simulink library "lib_Convection_NonDimParms"  (R2015a)
settings: Solver=ode45  StartTime=0.0  StopTime=10.0  RelTol=1e-3
settings Model: Creator=jlkratz  LastModifiedBy=jlkratz

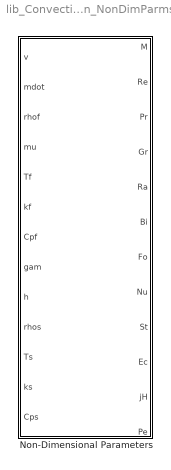
== system lib_Convection_NonDimParms ==
  Non-Dimensional Parameters : Subsystem  mask(TSAT: Non-Dimensional Parameters Block){M_M=on, Re_M=on, Pr_M=on, Gr_M=on, Ra_M=on, Bi_M=on, Fo_M=on, Nu_M=on, St_M=on, Ec_M=on, jH_M=on, Pe_M=on, perfGas_M=on, R_M=1716, mdot_A_or_rhov_M=on, A_M=1, L_M=1, g_M=32.174, t_M=1, BN_M=double(gcb)}
      mask prompts: M_M "M_M - Mach Number"; Re_M "Re_M - Reynolds Number"; Pr_M "Pr_M - Prandtl Number"; Gr_M "Gr_M - Grashof Number"; Ra_M "Ra_M - Rayliegh Number"; Bi_M "Bi_M - Biot Number"; Fo_M "Fo_M - Fourier Number"; Nu_M "Nu_M - Nusselt Number"; St_M "St_M - Stanton Number"; Ec_M "Ec_M - Eckert Number"; jH_M "jH_M - Colburn j facotr"; Pe_M "Pe_M - Peclet Number"; perfGas_M "perfGas_M - Perfect gas?"; R_M "R_M - Real gas constant"; mdot_A_or_rhov_M "mdot_A_or_rhov_M - Compute Re using mass flow rate or velocity (checked mdot, unchecked v)?"; A_M "A_M - Flow area"; L_M "L_M - Characteristic length"; g_M "g_M - Acceleration due to gravity"; t_M "t_M - Charateristic time-scale"; BN_M "BN_M - Block Name"
      mask help:
      | This block computes various non-dimensional quanties that are related to heat transfer. See the block help menu for a full description of the non-dimensional parameters addressed in this block and definitions of all of the inputs and parameters.
      |
      | This block can accept inputs of any dimensions as long as they are all consistent. Any units can be used in the inputs and parameters as long as they are consistent and on a total scale (no relative values and no units of a non-total scale. Ex. no degrees Celsius and Farhenhiet).
      mask init:
      | % Setup inports ----------------------------------------------------------%
      | 
      | % Inport Numbers
      | n = 1; %first inport
      | 
      | % Velocity
      | if M_M == 1 || (Re_M == 1 && mdot_A_or_rhov_M == 0) || Pe_M == 1 || Ec_M == 1 || St_M == 1
      |     if strcmp(get_param([BN_M '/v'],'BlockType'),'Constant')
      |         MSK_ReplaceBlock_TSAT([BN_M '/v'],'built-in/Inport');
      |     end
      |     set_param([BN_M '/v'],'Port',num2str(n));
      |     n = n + 1;
      | else
      |     if strcmp(get_param([BN_M '/v'],'BlockType'),'Inport')
      |         MSK_ReplaceBlock_TSAT([BN_M '/v'],'built-in/Constant');
      |         set_param([BN_M '/v'],'Value','10');
      |     end
      | end
      | 
      | % Mass Flow Rate
      | if (Re_M == 1 && mdot_A_or_rhov_M == 1)
      |     if strcmp(get_param([BN_M '/mdot'],'BlockType'),'Constant')
      |         MSK_ReplaceBlock_TSAT([BN_M '/mdot'],'built-in/Inport');
      |     end
      |     set_param([BN_M '/mdot'],'Port',num2str(n));
      |     n = n + 1;
      | else
      |     if strcmp(get_param([BN_M '/mdot'],'BlockType'),'Inport')
      |         MSK_ReplaceBlock_TSAT([BN_M '/mdot'],'built-in/Constant');
      |         set_param([BN_M '/mdot'],'Value','1');
      |     end
      | end
      | 
      | % Density of fluid
      | if (Re_M == 1 && mdot_A_or_rhov_M == 0) || Pe_M == 1 || St_M == 1 || Gr_M == 1 || Ra_M == 1
      |     if strcmp(get_param([BN_M '/rhof'],'BlockType'),'Constant')
      |         MSK_ReplaceBlock_TSAT([BN_M '/rhof'],'built-in/Inport');
      |     end
      |     set_param([BN_M '/rhof'],'Port',num2str(n));
      |     n = n + 1;
      | else
      |     if strcmp(get_param([BN_M '/rhof'],'BlockType'),'Inport')
      |         MSK_ReplaceBlock_TSAT([BN_M '/rhof'],'built-in/Constant');
      |         set_param([BN_M '/rhof'],'Value','0.00237');
      |     end
      | end
      | 
      | % Viscosity
      | if Re_M == 1 || Pr_M == 1 || Gr_M == 1 || Ra_M == 1 || jH_M == 1
      |     if strcmp(get_param([BN_M '/mu'],'BlockType'),'Constant')
      |         MSK_ReplaceBlock_TSAT([BN_M '/mu'],'built-in/Inport');
      |     end
      |     set_param([BN_M '/mu'],'Port',num2str(n));
      |     n = n + 1;
      | else
      |     if strcmp(get_param([BN_M '/mu'],'BlockType'),'Inport')
      |         MSK_ReplaceBlock_TSAT([BN_M '/mu'],'built-in/Constant');
      |         set_param([BN_M '/mu'],'Value','0.0000005');
      |     end
      | end
      | 
      | % Temperature of fluid
      | if Gr_M == 1 || Ra_M == 1 || Ec_M == 1 || (M_M == 1 && perfGas_M == 1)
      |     if strcmp(get_param([BN_M '/Tf'],'BlockType'),'Constant')
      |         MSK_ReplaceBlock_TSAT([BN_M '/Tf'],'built-in/Inport');
      |     end
      |     set_param([BN_M '/Tf'],'Port',num2str(n));
      |     n = n + 1;
      | else
      |     if strcmp(get_param([BN_M '/Tf'],'BlockType'),'Inport')
      |         MSK_ReplaceBlock_TSAT([BN_M '/Tf'],'built-in/Constant');
      |         set_param([BN_M '/Tf'],'Value','0.0000005');
      |     end
      | end
      | 
      | % Thermal conductivity of fluid
      | if Pr_M == 1 || Nu_M == 1 || Pe_M == 1
      |     if strcmp(get_param([BN_M '/kf'],'BlockType'),'Constant')
      |         MSK_ReplaceBlock_TSAT([BN_M '/kf'],'built-in/Inport');
      |     end
      |     set_param([BN_M '/kf'],'Port',num2str(n));
      |     n = n + 1;
      | else
      |     if strcmp(get_param([BN_M '/kf'],'BlockType'),'Inport')
      |         MSK_ReplaceBlock_TSAT([BN_M '/kf'],'built-in/Constant');
      |         set_param([BN_M '/kf'],'Value','0.00000413');
      |     end
      | end
      | 
      | % Heat Capacity of fluid
      | if Pr_M == 1 || Ec_M == 1 || Pe_M == 1 || St_M == 1
      |     if strcmp(get_param([BN_M '/Cpf'],'BlockType'),'Constant')
      |         MSK_ReplaceBlock_TSAT([BN_M '/Cpf'],'built-in/Inport');
      |     end
      |     set_param([BN_M '/Cpf'],'Port',num2str(n));
      |     n = n + 1;
      | else
      |     if strcmp(get_param([BN_M '/Cpf'],'BlockType'),'Inport')
      |         MSK_ReplaceBlock_TSAT([BN_M '/Cpf'],'built-in/Constant');
      |         set_param([BN_M '/Cpf'],'Value','7.72');
      |     end
      | end
      | 
      | % Specific heat ratio
      | if (M_M == 1 && perfGas_M == 1)
      |     if strcmp(get_param([BN_M '/gam'],'BlockType'),'Constant')
      |         MSK_ReplaceBlock_TSAT([BN_M '/gam'],'built-in/Inport');
      |     end
      |     set_param([BN_M '/gam'],'Port',num2str(n));
      |     n = n + 1;
      | else
      |     if strcmp(get_param([BN_M '/gam'],'BlockType'),'Inport')
      |         MSK_ReplaceBlock_TSAT([BN_M '/gam'],'built-in/Constant');
      |         set_param([BN_M '/gam'],'Value','1.4');
      |     end
      | end
      | 
      | % Convective heat transfer coefficient
      | if Bi_M == 1 || Nu_M == 1 || St_M == 1
      |     if strcmp(get_param([BN_M '/h'],'BlockType'),'Constant')
      |         MSK_ReplaceBlock_TSAT([BN_M '/h'],'built-in/Inport');
      |     end
      |     set_param([BN_M '/h'],'Port',num2str(n));
      |     n = n + 1;
      | else
      |     if strcmp(get_param([BN_M '/h'],'BlockType'),'Inport')
      |         MSK_ReplaceBlock_TSAT([BN_M '/h'],'built-in/Constant');
      |         set_param([BN_M '/h'],'Value','0.003');
      |     end
      | end
      | 
      | % Speed of sound
      | if (M_M == 1 && perfGas_M == 0)
      |     if strcmp(get_param([BN_M '/a'],'BlockType'),'Constant')
      |         MSK_ReplaceBlock_TSAT([BN_M '/a'],'built-in/Inport');
      |     end
      |     set_param([BN_M '/a'],'Port',num2str(n));
      |     n = n + 1;
      | else
      |     if strcmp(get_param([BN_M '/a'],'BlockType'),'Inport')
      |         MSK_ReplaceBlock_TSAT([BN_M '/a'],'built-in/Constant');
      |         set_param([BN_M '/a'],'Value','1125.33');
      |     end
      | end
      | 
      | % Expansion coefficient
      | if (Gr_M == 1 && perfGas_M == 0) || (Ra_M == 1 && perfGas_M == 0)
      |     if strcmp(get_param([BN_M '/beta'],'BlockType'),'Constant')
      |         MSK_ReplaceBlock_TSAT([BN_M '/beta'],'built-in/Inport');
      |     end
      |     set_param([BN_M '/beta'],'Port',num2str(n));
      |     n = n + 1;
      | else
      |     if strcmp(get_param([BN_M '/beta'],'BlockType'),'Inport')
      |         MSK_ReplaceBlock_TSAT([BN_M '/beta'],'built-in/Constant');
      |         set_param([BN_M '/beta'],'Value','0.002');
      |     end
      | end
      | 
      | % Density of solid (body)
      | if Fo_M == 1
      |     if strcmp(get_param([BN_M '/rhos'],'BlockType'),'Constant')
      |         MSK_ReplaceBlock_TSAT([BN_M '/rhos'],'built-in/Inport');
      |     end
      |     set_param([BN_M '/rhos'],'Port',num2str(n));
      |     n = n + 1;
      | else
      |     if strcmp(get_param([BN_M '/rhos'],'BlockType'),'Inport')
      |         MSK_ReplaceBlock_TSAT([BN_M '/rhos'],'built-in/Constant');
      |         set_param([BN_M '/rhos'],'Value','2');
      |     end
      | end
      | 
      | % Temperature of solid (body)
      | if Gr_M == 1 || Ra_M == 1 || Ec_M == 1
      |     if strcmp(get_param([BN_M '/Ts'],'BlockType'),'Constant')
      |         MSK_ReplaceBlock_TSAT([BN_M '/Ts'],'built-in/Inport');
      |     end
      |     set_param([BN_M '/Ts'],'Port',num2str(n));
      |     n = n + 1;
      | else
      |     if strcmp(get_param([BN_M '/Ts'],'BlockType'),'Inport')
      |         MSK_ReplaceBlock_TSAT([BN_M '/Ts'],'built-in/Constant');
      |         set_param([BN_M '/Ts'],'Value','1000');
      |     end
      | end
      | 
      | % Thermal conductivity of solid (body)
      | if Fo_M == 1 || Bi_M == 1
      |     if strcmp(get_param([BN_M '/ks'],'BlockType'),'Constant')
      |         MSK_ReplaceBlock_TSAT([BN_M '/ks'],'built-in/Inport');
      |     end
      |     set_param([BN_M '/ks'],'Port',num2str(n));
      |     n = n + 1;
      | else
      |     if strcmp(get_param([BN_M '/ks'],'BlockType'),'Inport')
      |         MSK_ReplaceBlock_TSAT([BN_M '/ks'],'built-in/Constant');
      |         set_param([BN_M '/ks'],'Value','0.005');
      |     end
      | end
      | 
      | % Heat Capacity of solid (body)
      | if Fo_M == 1
      |     if strcmp(get_param([BN_M '/Cps'],'BlockType'),'Constant')
      |         MSK_ReplaceBlock_TSAT([BN_M '/Cps'],'built-in/Inport');
      |     end
      |     set_param([BN_M '/Cps'],'Port',num2str(n));
      |     n = n + 1;
      | else
      |     if strcmp(get_param([BN_M '/Cps'],'BlockType'),'Inport')
      |         MSK_ReplaceBlock_TSAT([BN_M '/Cps'],'built-in/Constant');
      |         set_param([BN_M '/Cps'],'Value','3.2');
      |     end
      | end
      | 
      | %Setup outports ----------------------------------------------------------%
      | 
      | % Outport Numbers
      | N = 1; %first outport
      | 
      | % Mach number
      | if M_M == 1
      |     if strcmp(get_param([BN_M '/M'],'BlockType'),'Terminator')
      |         MSK_ReplaceBlock_TSAT([BN_M '/M'],'built-in/Outport');
      |     end
      |     set_param([BN_M '/M'],'Port',num2str(N));
      |     N = N + 1;
      | elseif M_M == 0
      |     if strcmp(get_param([BN_M '/M'],'BlockType'),'Outport')
      |         MSK_ReplaceBlock_TSAT([BN_M '/M'],'built-in/Terminator');
      |     end
      | end
      | 
      | % Reynolds number
      | if Re_M == 1
      |     if strcmp(get_param([BN_M '/Re'],'BlockType'),'Terminator')
      |         MSK_ReplaceBlock_TSAT([BN_M '/Re'],'built-in/Outport');
      |     end
      |     set_param([BN_M '/Re'],'Port',num2str(N));
      |     N = N + 1;
      | elseif Re_M == 0
      |     if strcmp(get_param([BN_M '/Re'],'BlockType'),'Outport')
      |         MSK_ReplaceBlock_TSAT([BN_M '/Re'],'built-in/Terminator');
      |     end
      | end
      | 
      | % Prantdl number
      | if Pr_M == 1
      |     if strcmp(get_param([BN_M '/Pr'],'BlockType'),'Terminator')
      |         MSK_ReplaceBlock_TSAT([BN_M '/Pr'],'built-in/Outport');
      |     end
      |     set_param([BN_M '/Pr'],'Port',num2str(N));
      |     N = N + 1;
      | elseif Pr_M == 0
      |     if strcmp(get_param([BN_M '/Pr'],'BlockType'),'Outport')
      |         MSK_ReplaceBlock_TSAT([BN_M '/Pr'],'built-in/Terminator');
      |     end
      | end
      | 
      | % Grashof number
      | if Gr_M == 1
      |     if strcmp(get_param([BN_M '/Gr'],'BlockType'),'Terminator')
      |         MSK_ReplaceBlock_TSAT([BN_M '/Gr'],'built-in/Outport');
      |     end
      |     set_param([BN_M '/Gr'],'Port',num2str(N));
      |     N = N + 1;
      | elseif Gr_M == 0
      |     if strcmp(get_param([BN_M '/Gr'],'BlockType'),'Outport')
      |         MSK_ReplaceBlock_TSAT([BN_M '/Gr'],'built-in/Terminator');
      |     end
      | end
      | 
      | % Rayliegh number
      | if Ra_M == 1
      |     if strcmp(get_param([BN_M '/Ra'],'BlockType'),'Terminator')
      |         MSK_ReplaceBlock_TSAT([BN_M '/Ra'],'built-in/Outport');
      |     end
      |     set_param([BN_M '/Ra'],'Port',num2str(N));
      |     N = N + 1;
      | elseif Ra_M == 0
      |     if strcmp(get_param([BN_M '/Ra'],'BlockType'),'Outport')
      |         MSK_ReplaceBlock_TSAT([BN_M '/Ra'],'built-in/Terminator');
      |     end
      | end
      | 
      | % Biot number
      | if Bi_M == 1
      |     if strcmp(get_param([BN_M '/Bi'],'BlockType'),'Terminator')
      |         MSK_ReplaceBlock_TSAT([BN_M '/Bi'],'built-in/Outport');
      |     end
      |     set_param([BN_M '/Bi'],'Port',num2str(N));
      |     N = N + 1;
      | elseif Bi_M == 0
      |     if strcmp(get_param([BN_M '/Bi'],'BlockType'),'Outport')
      |         MSK_ReplaceBlock_TSAT([BN_M '/Bi'],'built-in/Terminator');
      |     end
      | end
      | 
      | % Fourier number
      | if Fo_M == 1
      |     if strcmp(get_param([BN_M '/Fo'],'BlockType'),'Terminator')
      |         MSK_ReplaceBlock_TSAT([BN_M '/Fo'],'built-in/Outport');
      |     end
      |     set_param([BN_M '/Fo'],'Port',num2str(N));
      |     N = N + 1;
      | elseif Fo_M == 0
      |     if strcmp(get_param([BN_M '/Fo'],'BlockType'),'Outport')
      |         MSK_ReplaceBlock_TSAT([BN_M '/Fo'],'built-in/Terminator');
      |     end
      | end
      | 
      | % Nusselt Number
      | if Nu_M == 1
      |     if strcmp(get_param([BN_M '/Nu'],'BlockType'),'Terminator')
      |         MSK_ReplaceBlock_TSAT([BN_M '/Nu'],'built-in/Outport');
      |     end
      |     set_param([BN_M '/Nu'],'Port',num2str(N));
      |     N = N + 1;
      | elseif Nu_M == 0
      |     if strcmp(get_param([BN_M '/Nu'],'BlockType'),'Outport')
      |         MSK_ReplaceBlock_TSAT([BN_M '/Nu'],'built-in/Terminator');
      |     end
      | end
      | 
      | % Stanton Number
      | if St_M == 1
      |     if strcmp(get_param([BN_M '/St'],'BlockType'),'Terminator')
      |         MSK_ReplaceBlock_TSAT([BN_M '/St'],'built-in/Outport');
      |     end
      |     set_param([BN_M '/St'],'Port',num2str(N));
      |     N = N + 1;
      | elseif St_M == 0
      |     if strcmp(get_param([BN_M '/St'],'BlockType'),'Outport')
      |         MSK_ReplaceBlock_TSAT([BN_M '/St'],'built-in/Terminator');
      |     end
      | end
      | 
      | % Eckert Number
      | if Ec_M == 1
      |     if strcmp(get_param([BN_M '/Ec'],'BlockType'),'Terminator')
      |         MSK_ReplaceBlock_TSAT([BN_M '/Ec'],'built-in/Outport');
      |     end
      |     set_param([BN_M '/Ec'],'Port',num2str(N));
      |     N = N + 1;
      | elseif Ec_M == 0
      |     if strcmp(get_param([BN_M '/Ec'],'BlockType'),'Outport')
      |         MSK_ReplaceBlock_TSAT([BN_M '/Ec'],'built-in/Terminator');
      |     end
      | end
      | 
      | % Colburn j factor
      | if jH_M == 1
      |     if strcmp(get_param([BN_M '/jH'],'BlockType'),'Terminator')
      |         MSK_ReplaceBlock_TSAT([BN_M '/jH'],'built-in/Outport');
      |     end
      |     set_param([BN_M '/jH'],'Port',num2str(N));
      |     N = N + 1;
      | elseif jH_M == 0
      |     if strcmp(get_param([BN_M '/jH'],'BlockType'),'Outport')
      |         MSK_ReplaceBlock_TSAT([BN_M '/jH'],'built-in/Terminator');
      |     end
      | end
      | 
      | % Peclet number
      | if Pe_M == 1
      |     if strcmp(get_param([BN_M '/Pe'],'BlockType'),'Terminator')
      |         MSK_ReplaceBlock_TSAT([BN_M '/Pe'],'built-in/Outport');
      |     end
      |     set_param([BN_M '/Pe'],'Port',num2str(N));
      |     N = N + 1;
      | elseif Pe_M == 0
      |     if strcmp(get_param([BN_M '/Pe'],'BlockType'),'Outport')
      |         MSK_ReplaceBlock_TSAT([BN_M '/Pe'],'built-in/Terminator');
      |     end
      | end
      mask Help: web(which('Convection_TSAT_NonDimParams.html'),'-helpbrowser')
      mask Callback Re_M:
      | if length(get_param(gcb,'Gr_M')) == 2 || length(get_param(gcb,'Ra_M')) == 2 ...
      |         || length(get_param(gcb,'Bi_M')) == 2 || length(get_param(gcb,'Fo_M')) == 2 ...
      |         || length(get_param(gcb,'Nu_M')) == 2 || length(get_param(gcb,'Pe_M')) == 2
      |     %do nothing
      | else
      |     MSK_SEC_Enables2_TSAT('Re_M',17,'en')
      | end
      mask Callback Gr_M:
      | if length(get_param(gcb,'Ra_M')) ~= 2
      |     MSK_SEC_Enables2_TSAT('Gr_M',18,'en')
      | end
      | 
      | if length(get_param(gcb,'Re_M')) == 2 || length(get_param(gcb,'Ra_M')) == 2 ...
      |         || length(get_param(gcb,'Bi_M')) == 2 || length(get_param(gcb,'Fo_M')) == 2 ...
      |         || length(get_param(gcb,'Nu_M')) == 2 || length(get_param(gcb,'Pe_M')) == 2
      |     %do nothing
      | else
      |     MSK_SEC_Enables2_TSAT('Gr_M',17,'en')
      | end
      mask Callback Ra_M:
      | if length(get_param(gcb,'Gr_M')) ~= 2
      |     MSK_SEC_Enables2_TSAT('Ra_M',18,'en')
      | end
      | 
      | if length(get_param(gcb,'Gr_M')) == 2 || length(get_param(gcb,'Re_M')) == 2 ...
      |         || length(get_param(gcb,'Bi_M')) == 2 || length(get_param(gcb,'Fo_M')) == 2 ...
      |         || length(get_param(gcb,'Nu_M')) == 2 || length(get_param(gcb,'Pe_M')) == 2
      |     %do nothing
      | else
      |     MSK_SEC_Enables2_TSAT('Ra_M',17,'en')
      | end
      mask Callback Bi_M:
      | if length(get_param(gcb,'Gr_M')) == 2 || length(get_param(gcb,'Ra_M')) == 2 ...
      |         || length(get_param(gcb,'Re_M')) == 2 || length(get_param(gcb,'Fo_M')) == 2 ...
      |         || length(get_param(gcb,'Nu_M')) == 2 || length(get_param(gcb,'Pe_M')) == 2
      |     %do nothing
      | else
      |     MSK_SEC_Enables2_TSAT('Bi_M',17,'en')
      | end
      mask Callback Fo_M:
      | MSK_SEC_Enables_TSAT('Fo_M',19,'en')
      | 
      | if length(get_param(gcb,'Gr_M')) == 2 || length(get_param(gcb,'Ra_M')) == 2 ...
      |         || length(get_param(gcb,'Bi_M')) == 2 || length(get_param(gcb,'Re_M')) == 2 ...
      |         || length(get_param(gcb,'Nu_M')) == 2 || length(get_param(gcb,'Pe_M')) == 2
      |     %do nothing
      | else
      |     MSK_SEC_Enables2_TSAT('Fo_M',17,'en')
      | end
      mask Callback Nu_M:
      | if length(get_param(gcb,'Gr_M')) == 2 || length(get_param(gcb,'Ra_M')) == 2 ...
      |         || length(get_param(gcb,'Bi_M')) == 2 || length(get_param(gcb,'Fo_M')) == 2 ...
      |         || length(get_param(gcb,'Re_M')) == 2 || length(get_param(gcb,'Pe_M')) == 2
      |     %do nothing
      | else
      |     MSK_SEC_Enables2_TSAT('Nu_M',17,'en')
      | end
      mask Callback Pe_M:
      | if length(get_param(gcb,'Gr_M')) == 2 || length(get_param(gcb,'Ra_M')) == 2 ...
      |         || length(get_param(gcb,'Bi_M')) == 2 || length(get_param(gcb,'Fo_M')) == 2 ...
      |         || length(get_param(gcb,'Nu_M')) == 2 || length(get_param(gcb,'Re_M')) == 2
      |     %do nothing
      | else
      |     MSK_SEC_Enables2_TSAT('Pe_M',17,'en')
      | end
      mask Callback perfGas_M: MSK_SEC_Enables_TSAT('perfGas_M',14,'en')
      mask Callback mdot_A_or_rhov_M: MSK_SEC_Enables_TSAT('mdot_A_or_rhov_M',16,'en')
      mask DialogControl Container3 Prompt: Outputs
      mask DialogControl Container8 Prompt: Parameters

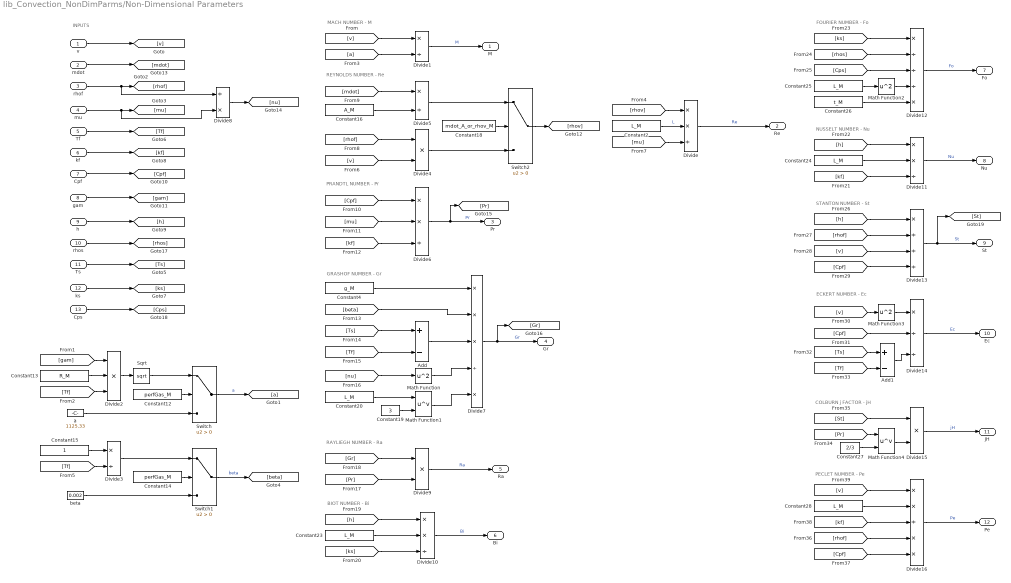
== system lib_Convection_NonDimParms/Non-Dimensional Parameters ==
  note: PECLET NUMBER - Pe
  note: STANTON NUMBER - St
  note: FOURIER NUMBER - Fo
  note: BIOT NUMBER - Bi
  note: MACH NUMBER - M
  note: REYNOLDS NUMBER - Re
  note: PRANDTL NUMBER - Pr
  note: GRASHOF NUMBER - Gr
  note: RAYLIEGH NUMBER - Ra
  note: NUSSELT NUMBER - Nu
  note: ECKERT NUMBER - Ec
  note: COLBURN j FACTOR - jH
  note: INPUTS
  v : Inport
  mdot : Inport  Port=2
  rhof : Inport  Port=3
  mu : Inport  Port=4
  Tf : Inport  Port=5
  kf : Inport  Port=6
  Cpf : Inport  Port=7
  gam : Inport  Port=8
  h : Inport  Port=9
  rhos : Inport  Port=10
  Ts : Inport  Port=11
  ks : Inport  Port=12
  Cps : Inport  Port=13
  Add : Sum  Inputs=+-
  Add1 : Sum  Inputs=+-
  Constant12 : Constant  Value=perfGas_M
  Constant13 : Constant  Value=R_M
  Constant14 : Constant  Value=perfGas_M
  Constant15 : Constant
  Constant16 : Constant  Value=A_M
  Constant18 : Constant  Value=mdot_A_or_rhov_M
  Constant19 : Constant  Value=3
  Constant{2,20,23..25,28} (6 alike) : Constant  Value=L_M
  Constant26 : Constant  Value=t_M
  Constant27 : Constant  Value=2/3
  Constant4 : Constant  Value=g_M
  Divide{,6,10..11} (4 alike) : Product  Inputs=**/
  Divide1 : Product  Inputs=*/
  Divide12 : Product  Inputs=*///*
  Divide13 : Product  Inputs=*///
  Divide14 : Product  Inputs=*//
  Divide15 : Product  Inputs=**
  Divide16 : Product  Inputs=**/**
  Divide2 : Product  Inputs=***
  Divide3 : Product  Inputs=*/
  Divide4 : Product  Inputs=**
  Divide5 : Product  Inputs=*/
  Divide7 : Product  Inputs=***/*
  Divide8 : Product  Inputs=/*
  Divide9 : Product  Inputs=**
  Math Function : Math  Operator=square  SaturateOnIntegerOverflow=on
  Math Function1 : Math  Operator=pow  SaturateOnIntegerOverflow=on
  Math Function2 : Math  Operator=square  SaturateOnIntegerOverflow=on
  Math Function3 : Math  Operator=square  SaturateOnIntegerOverflow=on
  Math Function4 : Math  Operator=pow  SaturateOnIntegerOverflow=on
  Sqrt : Sqrt  SaturateOnIntegerOverflow=on
  Switch : Switch  Criteria=u2 > Threshold
  Switch1 : Switch  Criteria=u2 > Threshold
  Switch2 : Switch  Criteria=u2 > Threshold
  a : Constant  Value=1125.33
  beta : Constant  Value=0.002
  M : Outport
  Re : Outport  Port=2
  Pr : Outport  Port=3
  Gr : Outport  Port=4
  Ra : Outport  Port=5
  Bi : Outport  Port=6
  Fo : Outport  Port=7
  Nu : Outport  Port=8
  St : Outport  Port=9
  Ec : Outport  Port=10
  jH : Outport  Port=11
  Pe : Outport  Port=12
  wires:
  Cps/1 -> [Cps]
  rhos/1 -> [rhos]
  [Pr] -> Math Function4/1
  [Cpf] -> Divide14/2
  Divide15/1 -> jH/1  "jH"
  Add1/1 -> Divide14/3
  Divide14/1 -> Ec/1  "Ec"
  [Ts] -> Add1/1
  Math Function3/1 -> Divide14/1
  [v] -> Math Function3/1
  [Tf] -> Add1/2
  [Cpf] -> Divide13/4
  Divide13/1 -> [St], St/1  "St"
  [v] -> Divide13/3
  [rhof] -> Divide13/2
  [h] -> Divide13/1
  Divide11/1 -> Nu/1  "Nu"
  [kf] -> Divide11/3
  Constant24/1 -> Divide11/2
  [h] -> Divide11/1
  Divide12/1 -> Fo/1  "Fo"
  [ks] -> Divide12/1
  [rhos] -> Divide12/2
  [Cps] -> Divide12/3
  Constant25/1 -> Math Function2/1
  Math Function2/1 -> Divide12/4
  Constant26/1 -> Divide12/5
  Constant23/1 -> Divide10/2
  [ks] -> Divide10/3
  Divide10/1 -> Bi/1  "Bi"
  [h] -> Divide10/1
  Divide9/1 -> Ra/1  "Ra"
  [Pr] -> Divide9/2
  [Gr] -> Divide9/1
  gam/1 -> [gam]
  Cpf/1 -> [Cpf]
  Divide8/1 -> [nu]
  Divide7/1 -> [Gr], Gr/1  "Gr"
  Math Function1/1 -> Divide7/5
  Math Function/1 -> Divide7/4
  Constant4/1 -> Divide7/1
  [beta] -> Divide7/2
  Add/1 -> Divide7/3
  Constant20/1 -> Math Function1/1
  [nu] -> Math Function/1
  Constant19/1 -> Math Function1/2
  [Tf] -> Add/2
  [Ts] -> Add/1
  Divide6/1 -> [Pr], Pr/1  "Pr"
  [kf] -> Divide6/3
  [mu] -> Divide6/2
  [Cpf] -> Divide6/1
  [mu] -> Divide/3
  Constant2/1 -> Divide/2  "L"
  [rhov] -> Divide/1
  Constant18/1 -> Switch2/2
  Switch2/1 -> [rhov]
  Divide5/1 -> Switch2/1
  Divide4/1 -> Switch2/3
  Constant16/1 -> Divide5/2
  [mdot] -> Divide5/1
  mdot/1 -> [mdot]
  [rhof] -> Divide4/1
  [v] -> Divide4/2
  Divide1/1 -> M/1  "M"
  mu/1 -> [mu], Divide8/2
  v/1 -> [v]
  rhof/1 -> [rhof], Divide8/1
  [a] -> Divide1/2
  [v] -> Divide1/1
  Switch1/1 -> [beta]  "beta"
  Switch/1 -> [a]  "a"
  Divide3/1 -> Switch1/1
  Constant15/1 -> Divide3/1
  [Tf] -> Divide3/2
  Constant14/1 -> Switch1/2
  Sqrt/1 -> Switch/1
  a/1 -> Switch/3
  Constant12/1 -> Switch/2
  [Tf] -> Divide2/3
  [gam] -> Divide2/1
  Constant13/1 -> Divide2/2
  Divide2/1 -> Sqrt/1
  kf/1 -> [kf]
  ks/1 -> [ks]
  h/1 -> [h]
  Tf/1 -> [Tf]
  Ts/1 -> [Ts]
  beta/1 -> Switch1/3
  Divide/1 -> Re/1  "Re"
  [St] -> Divide15/1
  Constant27/1 -> Math Function4/2
  Math Function4/1 -> Divide15/2
  [Cpf] -> Divide16/5
  [rhof] -> Divide16/4
  Constant28/1 -> Divide16/2
  [v] -> Divide16/1
  Divide16/1 -> Pe/1  "Pe"
  [kf] -> Divide16/3
